simulink model "modelo_esh"  (R2022b)
settings: Solver=ode45  StartTime=0.0  StopTime=1  RelTol=1e-3  EnableMultiTasking=on
values from neighbouring files (symbols this model uses):
  A = 4.91e-4    (= 0.000491)    [var_esh.m]
  C1 = 18.4    [var_esh.m]
  CL = 8.08    [var_es.m]    (also in var_esh.m)
  Cl = 2e-6    (= 2e-06)    [var_esh.m]
  K1 = 7.5e7    (= 75000000)    [var_esh.m]
  Ka = B*Vt    (= 31980)    [var_esh.m]
  Kc = 4e6    (= 4000000)    [var_esh.m]
  Kd = 0.007    [var_es.m]    (also in var_esh.m = 0.0575)
  Ki = 4.129    [var_es.m]    (also in var_esh.m = 4412.1219)
  KL = 3.3e9    (= 3300000000)    [var_es.m]    (also in var_esh.m)
  KP = 8.4e2    (= 840)    [var_esh.m]
  Kp = 2.915    [var_es.m]    (also in var_esh.m = 54.9946)
  Kv = 6.24e-5    (= 6.24e-05)    [var_esh.m]
  Kvp = 1    [var_esh.m]
  M = 1.261    [var_es.m]    (also in var_esh.m = 1.5)
libraries: slpidlib x1
settings Model: Creator=11802972  LastModifiedBy=andre
settings SolverCC: AlgebraicLoopSolver=TrustRegion
settings DataIOCC: LimitDataPoints=on  SaveFormat=Array  ReturnWorkspaceOutputs=off
settings OptimizationCC: LifeSpan=inf
settings DebuggingCC: UnconnectedInputMsg=warning  UnconnectedOutputMsg=warning  UnconnectedLineMsg=warning  SFUnexpectedBacktrackingDiag=warning  SFNoUnconditionalDefaultTransitionDiag=warning  SFExecutionAtInitializationDiag=none  SFMachineParentedDataDiag=warning  ArithmeticOperatorsInVariantConditions=warning
settings HardwareCC: ProdBitPerPointer=32  ProdBitPerSizeT=32  ProdBitPerPtrDiffT=32  ProdLargestAtomicFloat=None  ProdIntDivRoundTo=Undefined  ProdEndianess=Unspecified  ProdWordSize=32  ProdHWDeviceType=32-bit Generic
settings ModelReferenceCC: PropagateSignalLabelsOutOfModel=off
settings SFSimCC: SimUseLocalCustomCode=off  CustomCodeUndefinedFunction=UseInterfaceOnly
settings RTWCC: RTWUseLocalCustomCode=off
settings CodeAppCC: StateflowObjectComments=on
settings GRTTargetCC: TargetLangStandard=C89/C90 (ANSI)
settings ConfigComp: CovMetricSettings=dw  CovSaveCumulativeToWorkspaceVar=on  CovSaveSingleToWorkspaceVar=on  CovExternalEMLEnable=off

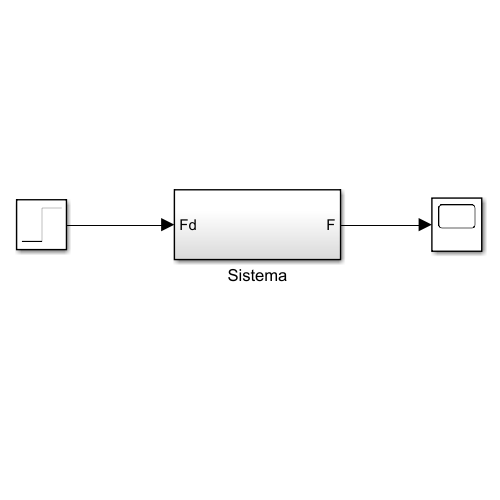
[thumbnail: Simulink's stored preview of the top-level diagram]
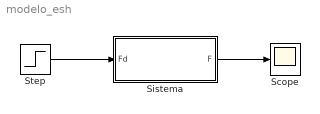
== system modelo_esh ==
  Scope : Scope
  "Sistema " : Subsystem
  Step : Step  Time=0  SampleTime=0
  wires:
  "Sistema "/1(F) -> Scope/1
  Step/1 -> "Sistema "/1(Fd)

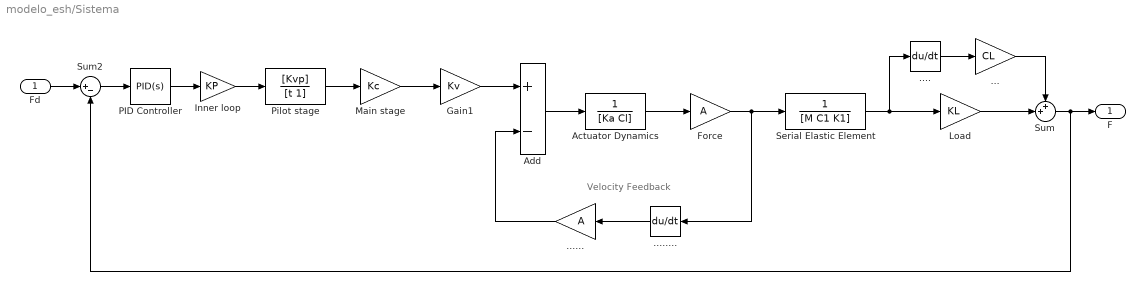
== system modelo_esh/Sistema  ==
  note: Velocity Feedback
  Fd : Inport
  ... : Gain  Gain=CL
  .... : Derivative
  ...... : Gain  Gain=A
  ........ : Derivative
  Actuator Dynamics : TransferFcn  Denominator=[Ka Cl]
  Add : Sum  Inputs=+-
  Force : Gain  Gain=A
  Gain1 : Gain  Gain=Kv
  Inner loop : Gain  Gain=KP
  Load : Gain  Gain=KL
  Main stage : Gain  Gain=Kc
  PID Controller : slpidlib/PID Controller  Controller=PID  Form=Parallel  TimeDomain=Continuous-time  UseExternalTs=off  SampleTime=-1  IntegratorMethod=Forward Euler  FilterMethod=Forward Euler  ControllerParametersSource=internal  P=Kp  I=Ki  UseKiTs=off  D=Kd  N=100  UseFilter=on  TunerSelectOption=Transfer Function Based (PID Tuner App)  InitialConditionSource=internal  InitialConditionForIntegrator=0  InitialConditionForFilter=0  DifferentiatorICPrevScaledInput=0  ExternalReset=none  TrackingMode=off  Kt=1  LimitOutput=off  SatLimitsSource=internal  UpperSaturationLimit=inf  LowerSaturationLimit=-inf  LinearizeAsGain=on  AntiWindupMode=none  Kb=1  LimitIntegrator=off  UpperIntegratorSaturationLimit=inf  LowerIntegratorSaturationLimit=-inf  POutMin=[]  POutMax=[]  IOutMin=[]  IOutMax=[]  DOutMin=[]  DOutMax=[]  NOutMin=[]  NOutMax=[]  SumOutMin=[]  SumOutMax=[]  SaturationOutMin=[]  SaturationOutMax=[]  PParamMin=[]  PParamMax=[]  IParamMin=[]  IParamMax=[]  DParamMin=[]  DParamMax=[]  NParamMin=[]  NParamMax=[]  KbParamMin=[]  KbParamMax=[]  KtParamMin=[]  KtParamMax=[]  KbOutMin=[]  KbOutMax=[]  KtOutMin=[]  KtOutMax=[]  IntegratorOutMin=[]  IntegratorOutMax=[]  FilterOutMin=[]  FilterOutMax=[]  SumI1OutMin=[]  SumI1OutMax=[]  SumI2OutMin=[]  SumI2OutMax=[]  SumI3OutMin=[]  SumI3OutMax=[]  SumI4OutMin=[]  SumI4OutMax=[]  SumDOutMin=[]  SumDOutMax=[]  DifferentiatorOutMin=[]  DifferentiatorOutMax=[]  FilterDiffOutCoefMin=[]  FilterDiffOutCoefMax=[]  ReciprocalOutMin=[]  ReciprocalOutMax=[]  SumDenOutMin=[]  SumDenOutMax=[]  SumNumOutMin=[]  SumNumOutMax=[]  DivideOutMin=[]  DivideOutMax=[]  UdiffTsProdOutMin=[]  UdiffTsProdOutMax=[]  NTsProdOutMin=[]  NTsProdOutMax=[]  UintegralTsProdOutMin=[]  UintegralTsProdOutMax=[]  UngainTsProdOutMin=[]  UngainTsProdOutMax=[]  ClampingZeroOutDataTypeStr=Inherit: Inherit via back propagation  ClampingZeroOutMin=[]  ClampingZeroOutMax=[]  FilterDenConstantOutDataTypeStr=Inherit: Inherit via back propagation  FilterDenConstantOutMin=[]  FilterDenConstantOutMax=[]  PCopyOutDataTypeStr=Inherit: Inherit via back propagation  PCopyOutMin=[]  PCopyOutMax=[]  NCopyOutDataTypeStr=Inherit: Inherit via back propagation  NCopyOutMin=[]  NCopyOutMax=[]  IntegratorContinuousStateAttributes=''  IntegratorStateMustResolveToSignalObject=off  IntegratorRTWStateStorageClass=Auto  FilterContinuousStateAttributes=''  FilterStateMustResolveToSignalObject=off  FilterRTWStateStorageClass=Auto  ParallelPVariant=InternalParameters  IdealPVariant=Disabled  IVariant=InternalParameters  DVariant=InternalParameters  IntegratorVariant=Continuous  SatVariant=Disabled  AWVariant=Passthrough  PCopyVariant=Disabled  TRVariant=Disabled  FdbkBlocksVariant=Forward  IdealPFdbkVariant=Disabled  SatFdbkVariant=Disabled  DerivativeFilterVariant=ContFilter  NVariant=InternalParameters  NCopyVariant=Disabled  FilterICVariant=InternalICsFilter  IntegratorICVariant=InternalICs  ExternalResetVariant=Disabled  TRSumVariant=Passthrough  SumFdbkVariant=Disabled  SumVariant=Sum_PID  TsampFilterVariant=InternalTs  TsampNgainVariant=Passthrough  TsampIntegralVariant=Passthrough  ExternalSaturationOutDataTypeStr=Inherit: Same as second input
  Pilot stage : TransferFcn  Numerator=[Kvp]  Denominator=[t 1]
  Serial Elastic Element : TransferFcn  Denominator=[M C1 K1]
  Sum : Sum  Inputs=++|
  Sum2 : Sum  Inputs=|+-
  F : Outport
  wires:
  Fd/1 -> Sum2/1
  Sum2/1 -> PID Controller/1
  PID Controller/1 -> Inner loop/1
  Inner loop/1 -> Pilot stage/1
  Pilot stage/1 -> Main stage/1
  Main stage/1 -> Gain1/1
  Gain1/1 -> Add/1
  Add/1 -> Actuator Dynamics/1
  Actuator Dynamics/1 -> Force/1
  ....../1 -> Add/2
  ......../1 -> ....../1
  Force/1 -> Serial Elastic Element/1, ......../1
  ..../1 -> .../1
  Serial Elastic Element/1 -> ..../1, Load/1
  Load/1 -> Sum/2
  .../1 -> Sum/1
  Sum/1 -> Sum2/2, F/1
